simulink model "tractor"  (R2018a)
settings: Solver=VariableStepAuto  StartTime=0.0  StopTime=0.1  RelTol=1e-3
values from neighbouring files (symbols this model uses):
  etheta = abs(etheta)    [speed_test.m]
  fait = fait1(i)    [speed_test.m]
  speed = 0.8    [speed_test.m]
  thetat = theta1(i)    [speed_test.m]
  vtheta = -0.2356    [speed_test.m]
  xt = xt1(i)    [speed_test.m]
  yt = yt1(i)    [speed_test.m]
settings Model: Creator=18428  LastModifiedBy=Administrator

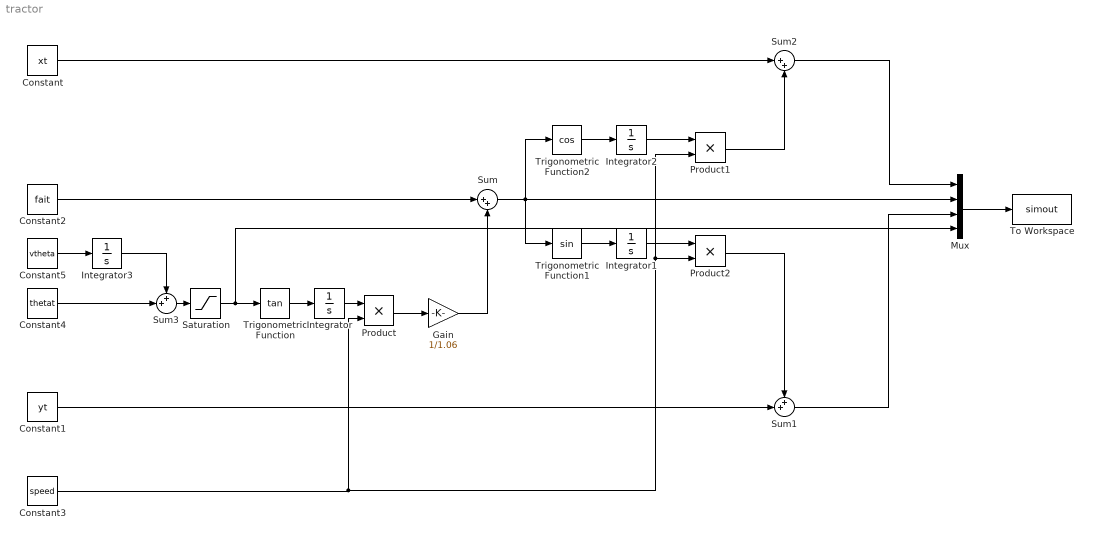
== system tractor ==
  Constant : Constant  Value=xt
  Constant1 : Constant  Value=yt
  Constant2 : Constant  Value=fait
  Constant3 : Constant  Value=speed
  Constant4 : Constant  Value=thetat
  Constant5 : Constant  Value=vtheta
  Gain : Gain  Gain=1/1.06
  Integrator{,1..3} (4 alike) : Integrator
  Mux : Mux
  Product : Product
  Product1 : Product
  Product2 : Product
  Saturation : Saturate  UpperLimit=etheta  LowerLimit=-etheta
  Sum : Sum  Inputs=|++
  Sum1 : Sum  Inputs=++|
  Sum2 : Sum  Inputs=|++
  Sum3 : Sum  Inputs=++|
  To Workspace : ToWorkspace  VariableName=simout  SaveFormat=Timeseries  SampleTime=-1
  Trigonometric Function : Trigonometry  Operator=tan
  Trigonometric Function1 : Trigonometry
  Trigonometric Function2 : Trigonometry  Operator=cos
  wires:
  Constant2/1 -> Sum/1
  Constant4/1 -> Sum3/2
  Trigonometric Function/1 -> Integrator/1
  Constant1/1 -> Sum1/2
  Sum/1 -> Mux/2, Trigonometric Function1/1, Trigonometric Function2/1
  Trigonometric Function1/1 -> Integrator1/1
  Trigonometric Function2/1 -> Integrator2/1
  Constant/1 -> Sum2/1
  Sum2/1 -> Mux/1
  Mux/1 -> To Workspace/1
  Sum1/1 -> Mux/3
  Constant3/1 -> Product2/2, Product1/2, Product/2
  Sum3/1 -> Saturation/1
  Saturation/1 -> Mux/4, Trigonometric Function/1
  Integrator/1 -> Product/1
  Product/1 -> Gain/1
  Gain/1 -> Sum/2
  Integrator2/1 -> Product1/1
  Integrator1/1 -> Product2/1
  Product1/1 -> Sum2/2
  Product2/1 -> Sum1/1
  Constant5/1 -> Integrator3/1
  Integrator3/1 -> Sum3/1
